simulink model "MdXX_Rsp"  (R2018b)
settings: Solver=FixedStepDiscrete  StartTime=0.0  StopTime=10.0  FixedStep=0.01  RelTol=1e-3
settings Model: Creator=sn2xws  LastModifiedBy=sn2xws
settings DataIOCC: SaveFormat=StructureWithTime
settings OptimizationCC: DefaultParameterBehavior=Inlined  EnhancedBackFolding=on  PassReuseOutputArgsAs=Individual arguments  ZeroExternalMemoryAtStartup=off  ZeroInternalMemoryAtStartup=off  OptimizeBlockOrder=speed  DifferentSizesBufferReuse=on  OptimizationCustomize=off
settings DebuggingCC: ParameterTunabilityLossMsg=error
settings ModelReferenceCC: ModelReferenceNumInstancesAllowed=Single
settings SFSimCC: MATLABDynamicMemAlloc=off
settings RTWCC: SystemTargetFile=autosar.tlc  GenCodeOnly=on  TemplateMakefile=ert_default_tmf  Description=AUTOSAR  GenerateReport=on  IncludeHyperlinkInReport=on  LaunchReport=on  GenerateTraceInfo=on  GenerateTraceReport=on  GenerateTraceReportSl=on  GenerateTraceReportSf=on  GenerateTraceReportEml=on
settings CodeAppCC: ForceParamTrailComments=on  IgnoreCustomStorageClasses=off  OperatorAnnotations=on  SimulinkDataObjDesc=on  SFDataObjDesc=on  InsertBlockDesc=on
settings STFCustomTargetCC: TargetLangStandard=C99 (ISO)  MultiwordLength=256  ParMdlRefBuildCompliant=on  CompOptLevelCompliant=on  IncludeMdlTerminateFcn=off  CombineOutputUpdateFcns=on  SuppressErrorStatus=on  ERTCustomFileBanners=on  SupportNonFinite=off  SupportComplex=off  SupportContinuousTime=off  SupportNonInlinedSFcns=off  RemoveResetFunc=on  MATLABClassNameForMDSCustomization=Simulink.SoftwareTarget.ERTCustomization  AutosarCompliant=on  UseToolchainInfoCompliant=on  LookupTableObjectStructAxisOrder=2,1,3,4,...  LUTObjectStructOrderEvenSpacing=Size,Table,Breakpoints  SystemTargetFile=autosar.tlc
settings ERTTargetCC: TargetLangStandard=C99 (ISO)  ConcurrentExecutionCompliant=off  IncludeMdlTerminateFcn=off  SuppressErrorStatus=on  SupportNonFinite=off  SupportComplex=off  ModelStepFunctionPrototypeControlCompliant=off  CPPClassGenCompliant=off  AutosarCompliant=on  LookupTableObjectStructAxisOrder=2,1,3,4,...  LUTObjectStructOrderEvenSpacing=Size,Table,Breakpoints  InlinedParameterPlacement=NonHierarchical  ERTCustomFileTemplate=example_file_process.tlc

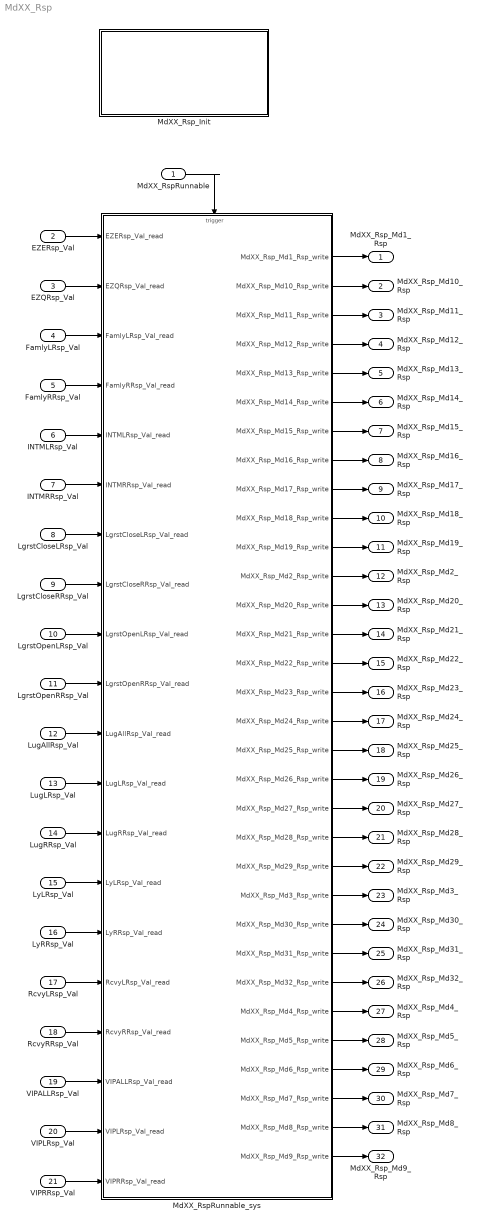
== system MdXX_Rsp ==
  MdXX_RspRunnable : Inport  SampleTime=0.01  OutputFunctionCall=on
  EZERsp_Val : Inport  Port=2  OutDataTypeStr=Enum: MdRspLocal1  PortDimensions=1
  EZQRsp_Val : Inport  Port=3  OutDataTypeStr=Enum: MdRspLocal1  PortDimensions=1
  FamlyLRsp_Val : Inport  Port=4  OutDataTypeStr=Enum: MdRspLocal1  PortDimensions=1
  FamlyRRsp_Val : Inport  Port=5  OutDataTypeStr=Enum: MdRspLocal1  PortDimensions=1
  INTMLRsp_Val : Inport  Port=6  OutDataTypeStr=Enum: MdRspLocal1  PortDimensions=1
  INTMRRsp_Val : Inport  Port=7  OutDataTypeStr=Enum: MdRspLocal1  PortDimensions=1
  LgrstCloseLRsp_Val : Inport  Port=8  OutDataTypeStr=Enum: MdRspLocal1  PortDimensions=1
  LgrstCloseRRsp_Val : Inport  Port=9  OutDataTypeStr=Enum: MdRspLocal1  PortDimensions=1
  LgrstOpenLRsp_Val : Inport  Port=10  OutDataTypeStr=Enum: MdRspLocal1  PortDimensions=1
  LgrstOpenRRsp_Val : Inport  Port=11  OutDataTypeStr=Enum: MdRspLocal1  PortDimensions=1
  LugAllRsp_Val : Inport  Port=12  OutDataTypeStr=Enum: MdRspLocal1  PortDimensions=1
  LugLRsp_Val : Inport  Port=13  OutDataTypeStr=Enum: MdRspLocal1  PortDimensions=1
  LugRRsp_Val : Inport  Port=14  OutDataTypeStr=Enum: MdRspLocal1  PortDimensions=1
  LyLRsp_Val : Inport  Port=15  OutDataTypeStr=Enum: MdRspLocal1  PortDimensions=1
  LyRRsp_Val : Inport  Port=16  OutDataTypeStr=Enum: MdRspLocal1  PortDimensions=1
  RcvyLRsp_Val : Inport  Port=17  OutDataTypeStr=Enum: MdRspLocal1  PortDimensions=1
  RcvyRRsp_Val : Inport  Port=18  OutDataTypeStr=Enum: MdRspLocal1  PortDimensions=1
  VIPALLRsp_Val : Inport  Port=19  OutDataTypeStr=Enum: MdRspLocal1  PortDimensions=1
  VIPLRsp_Val : Inport  Port=20  OutDataTypeStr=Enum: MdRspLocal1  PortDimensions=1
  VIPRRsp_Val : Inport  Port=21  OutDataTypeStr=Enum: MdRspLocal1  PortDimensions=1
  MdXX_RspRunnable_sys : Subsystem
  MdXX_Rsp_Init : Subsystem
  MdXX_Rsp_Md1_Rsp : Outport  OutDataTypeStr=Enum: MdRspLocal1  PortDimensions=1
  MdXX_Rsp_Md10_Rsp : Outport  Port=2  OutDataTypeStr=Enum: MdRspLocal1  PortDimensions=1
  MdXX_Rsp_Md11_Rsp : Outport  Port=3  OutDataTypeStr=Enum: MdRspLocal1  PortDimensions=1
  MdXX_Rsp_Md12_Rsp : Outport  Port=4  OutDataTypeStr=Enum: MdRspLocal1  PortDimensions=1
  MdXX_Rsp_Md13_Rsp : Outport  Port=5  OutDataTypeStr=Enum: MdRspLocal1  PortDimensions=1
  MdXX_Rsp_Md14_Rsp : Outport  Port=6  OutDataTypeStr=Enum: MdRspLocal1  PortDimensions=1
  MdXX_Rsp_Md15_Rsp : Outport  Port=7  OutDataTypeStr=Enum: MdRspLocal1  PortDimensions=1
  MdXX_Rsp_Md16_Rsp : Outport  Port=8  OutDataTypeStr=Enum: MdRspLocal1  PortDimensions=1
  MdXX_Rsp_Md17_Rsp : Outport  Port=9  OutDataTypeStr=Enum: MdRspLocal1  PortDimensions=1
  MdXX_Rsp_Md18_Rsp : Outport  Port=10  OutDataTypeStr=Enum: MdRspLocal1  PortDimensions=1
  MdXX_Rsp_Md19_Rsp : Outport  Port=11  OutDataTypeStr=Enum: MdRspLocal1  PortDimensions=1
  MdXX_Rsp_Md2_Rsp : Outport  Port=12  OutDataTypeStr=Enum: MdRspLocal1  PortDimensions=1
  MdXX_Rsp_Md20_Rsp : Outport  Port=13  OutDataTypeStr=Enum: MdRspLocal1  PortDimensions=1
  MdXX_Rsp_Md21_Rsp : Outport  Port=14  OutDataTypeStr=Enum: MdRspLocal1  PortDimensions=1
  MdXX_Rsp_Md22_Rsp : Outport  Port=15  OutDataTypeStr=Enum: MdRspLocal1  PortDimensions=1
  MdXX_Rsp_Md23_Rsp : Outport  Port=16  OutDataTypeStr=Enum: MdRspLocal1  PortDimensions=1
  MdXX_Rsp_Md24_Rsp : Outport  Port=17  OutDataTypeStr=Enum: MdRspLocal1  PortDimensions=1
  MdXX_Rsp_Md25_Rsp : Outport  Port=18  OutDataTypeStr=Enum: MdRspLocal1  PortDimensions=1
  MdXX_Rsp_Md26_Rsp : Outport  Port=19  OutDataTypeStr=Enum: MdRspLocal1  PortDimensions=1
  MdXX_Rsp_Md27_Rsp : Outport  Port=20  OutDataTypeStr=Enum: MdRspLocal1  PortDimensions=1
  MdXX_Rsp_Md28_Rsp : Outport  Port=21  OutDataTypeStr=Enum: MdRspLocal1  PortDimensions=1
  MdXX_Rsp_Md29_Rsp : Outport  Port=22  OutDataTypeStr=Enum: MdRspLocal1  PortDimensions=1
  MdXX_Rsp_Md3_Rsp : Outport  Port=23  OutDataTypeStr=Enum: MdRspLocal1  PortDimensions=1
  MdXX_Rsp_Md30_Rsp : Outport  Port=24  OutDataTypeStr=Enum: MdRspLocal1  PortDimensions=1
  MdXX_Rsp_Md31_Rsp : Outport  Port=25  OutDataTypeStr=Enum: MdRspLocal1  PortDimensions=1
  MdXX_Rsp_Md32_Rsp : Outport  Port=26  OutDataTypeStr=Enum: MdRspLocal1  PortDimensions=1
  MdXX_Rsp_Md4_Rsp : Outport  Port=27  OutDataTypeStr=Enum: MdRspLocal1  PortDimensions=1
  MdXX_Rsp_Md5_Rsp : Outport  Port=28  OutDataTypeStr=Enum: MdRspLocal1  PortDimensions=1
  MdXX_Rsp_Md6_Rsp : Outport  Port=29  OutDataTypeStr=Enum: MdRspLocal1  PortDimensions=1
  MdXX_Rsp_Md7_Rsp : Outport  Port=30  OutDataTypeStr=Enum: MdRspLocal1  PortDimensions=1
  MdXX_Rsp_Md8_Rsp : Outport  Port=31  OutDataTypeStr=Enum: MdRspLocal1  PortDimensions=1
  MdXX_Rsp_Md9_Rsp : Outport  Port=32  OutDataTypeStr=Enum: MdRspLocal1  PortDimensions=1
  wires:
  EZERsp_Val/1 -> MdXX_RspRunnable_sys/1(EZERsp_Val_read)
  EZQRsp_Val/1 -> MdXX_RspRunnable_sys/2(EZQRsp_Val_read)
  FamlyLRsp_Val/1 -> MdXX_RspRunnable_sys/3(FamlyLRsp_Val_read)
  FamlyRRsp_Val/1 -> MdXX_RspRunnable_sys/4(FamlyRRsp_Val_read)
  INTMLRsp_Val/1 -> MdXX_RspRunnable_sys/5(INTMLRsp_Val_read)
  INTMRRsp_Val/1 -> MdXX_RspRunnable_sys/6(INTMRRsp_Val_read)
  LgrstCloseLRsp_Val/1 -> MdXX_RspRunnable_sys/7(LgrstCloseLRsp_Val_read)
  LgrstCloseRRsp_Val/1 -> MdXX_RspRunnable_sys/8(LgrstCloseRRsp_Val_read)
  LgrstOpenLRsp_Val/1 -> MdXX_RspRunnable_sys/9(LgrstOpenLRsp_Val_read)
  LgrstOpenRRsp_Val/1 -> MdXX_RspRunnable_sys/10(LgrstOpenRRsp_Val_read)
  LugAllRsp_Val/1 -> MdXX_RspRunnable_sys/11(LugAllRsp_Val_read)
  LugLRsp_Val/1 -> MdXX_RspRunnable_sys/12(LugLRsp_Val_read)
  LugRRsp_Val/1 -> MdXX_RspRunnable_sys/13(LugRRsp_Val_read)
  LyLRsp_Val/1 -> MdXX_RspRunnable_sys/14(LyLRsp_Val_read)
  LyRRsp_Val/1 -> MdXX_RspRunnable_sys/15(LyRRsp_Val_read)
  RcvyLRsp_Val/1 -> MdXX_RspRunnable_sys/16(RcvyLRsp_Val_read)
  RcvyRRsp_Val/1 -> MdXX_RspRunnable_sys/17(RcvyRRsp_Val_read)
  VIPALLRsp_Val/1 -> MdXX_RspRunnable_sys/18(VIPALLRsp_Val_read)
  VIPLRsp_Val/1 -> MdXX_RspRunnable_sys/19(VIPLRsp_Val_read)
  VIPRRsp_Val/1 -> MdXX_RspRunnable_sys/20(VIPRRsp_Val_read)
  MdXX_RspRunnable_sys/1(MdXX_Rsp_Md1_Rsp_write) -> MdXX_Rsp_Md1_Rsp/1
  MdXX_RspRunnable_sys/2(MdXX_Rsp_Md10_Rsp_write) -> MdXX_Rsp_Md10_Rsp/1
  MdXX_RspRunnable_sys/3(MdXX_Rsp_Md11_Rsp_write) -> MdXX_Rsp_Md11_Rsp/1
  MdXX_RspRunnable_sys/4(MdXX_Rsp_Md12_Rsp_write) -> MdXX_Rsp_Md12_Rsp/1
  MdXX_RspRunnable_sys/5(MdXX_Rsp_Md13_Rsp_write) -> MdXX_Rsp_Md13_Rsp/1
  MdXX_RspRunnable_sys/6(MdXX_Rsp_Md14_Rsp_write) -> MdXX_Rsp_Md14_Rsp/1
  MdXX_RspRunnable_sys/7(MdXX_Rsp_Md15_Rsp_write) -> MdXX_Rsp_Md15_Rsp/1
  MdXX_RspRunnable_sys/8(MdXX_Rsp_Md16_Rsp_write) -> MdXX_Rsp_Md16_Rsp/1
  MdXX_RspRunnable_sys/9(MdXX_Rsp_Md17_Rsp_write) -> MdXX_Rsp_Md17_Rsp/1
  MdXX_RspRunnable_sys/10(MdXX_Rsp_Md18_Rsp_write) -> MdXX_Rsp_Md18_Rsp/1
  MdXX_RspRunnable_sys/11(MdXX_Rsp_Md19_Rsp_write) -> MdXX_Rsp_Md19_Rsp/1
  MdXX_RspRunnable_sys/12(MdXX_Rsp_Md2_Rsp_write) -> MdXX_Rsp_Md2_Rsp/1
  MdXX_RspRunnable_sys/13(MdXX_Rsp_Md20_Rsp_write) -> MdXX_Rsp_Md20_Rsp/1
  MdXX_RspRunnable_sys/14(MdXX_Rsp_Md21_Rsp_write) -> MdXX_Rsp_Md21_Rsp/1
  MdXX_RspRunnable_sys/15(MdXX_Rsp_Md22_Rsp_write) -> MdXX_Rsp_Md22_Rsp/1
  MdXX_RspRunnable_sys/16(MdXX_Rsp_Md23_Rsp_write) -> MdXX_Rsp_Md23_Rsp/1
  MdXX_RspRunnable_sys/17(MdXX_Rsp_Md24_Rsp_write) -> MdXX_Rsp_Md24_Rsp/1
  MdXX_RspRunnable_sys/18(MdXX_Rsp_Md25_Rsp_write) -> MdXX_Rsp_Md25_Rsp/1
  MdXX_RspRunnable_sys/19(MdXX_Rsp_Md26_Rsp_write) -> MdXX_Rsp_Md26_Rsp/1
  MdXX_RspRunnable_sys/20(MdXX_Rsp_Md27_Rsp_write) -> MdXX_Rsp_Md27_Rsp/1
  MdXX_RspRunnable_sys/21(MdXX_Rsp_Md28_Rsp_write) -> MdXX_Rsp_Md28_Rsp/1
  MdXX_RspRunnable_sys/22(MdXX_Rsp_Md29_Rsp_write) -> MdXX_Rsp_Md29_Rsp/1
  MdXX_RspRunnable_sys/23(MdXX_Rsp_Md3_Rsp_write) -> MdXX_Rsp_Md3_Rsp/1
  MdXX_RspRunnable_sys/24(MdXX_Rsp_Md30_Rsp_write) -> MdXX_Rsp_Md30_Rsp/1
  MdXX_RspRunnable_sys/25(MdXX_Rsp_Md31_Rsp_write) -> MdXX_Rsp_Md31_Rsp/1
  MdXX_RspRunnable_sys/26(MdXX_Rsp_Md32_Rsp_write) -> MdXX_Rsp_Md32_Rsp/1
  MdXX_RspRunnable_sys/27(MdXX_Rsp_Md4_Rsp_write) -> MdXX_Rsp_Md4_Rsp/1
  MdXX_RspRunnable_sys/28(MdXX_Rsp_Md5_Rsp_write) -> MdXX_Rsp_Md5_Rsp/1
  MdXX_RspRunnable_sys/29(MdXX_Rsp_Md6_Rsp_write) -> MdXX_Rsp_Md6_Rsp/1
  MdXX_RspRunnable_sys/30(MdXX_Rsp_Md7_Rsp_write) -> MdXX_Rsp_Md7_Rsp/1
  MdXX_RspRunnable_sys/31(MdXX_Rsp_Md8_Rsp_write) -> MdXX_Rsp_Md8_Rsp/1
  MdXX_RspRunnable_sys/32(MdXX_Rsp_Md9_Rsp_write) -> MdXX_Rsp_Md9_Rsp/1
  MdXX_RspRunnable/1 -> MdXX_RspRunnable_sys/Trigger

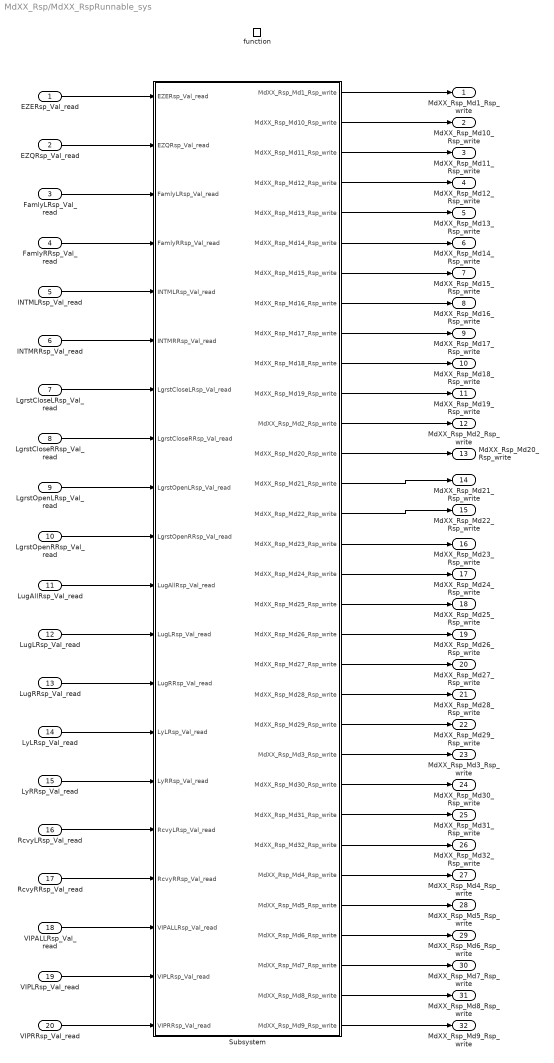
== system MdXX_Rsp/MdXX_RspRunnable_sys ==
  EZERsp_Val_read : Inport
  EZQRsp_Val_read : Inport  Port=2
  FamlyLRsp_Val_read : Inport  Port=3
  FamlyRRsp_Val_read : Inport  Port=4
  INTMLRsp_Val_read : Inport  Port=5
  INTMRRsp_Val_read : Inport  Port=6
  LgrstCloseLRsp_Val_read : Inport  Port=7
  LgrstCloseRRsp_Val_read : Inport  Port=8
  LgrstOpenLRsp_Val_read : Inport  Port=9
  LgrstOpenRRsp_Val_read : Inport  Port=10
  LugAllRsp_Val_read : Inport  Port=11
  LugLRsp_Val_read : Inport  Port=12
  LugRRsp_Val_read : Inport  Port=13
  LyLRsp_Val_read : Inport  Port=14
  LyRRsp_Val_read : Inport  Port=15
  RcvyLRsp_Val_read : Inport  Port=16
  RcvyRRsp_Val_read : Inport  Port=17
  VIPALLRsp_Val_read : Inport  Port=18
  VIPLRsp_Val_read : Inport  Port=19
  VIPRRsp_Val_read : Inport  Port=20
  function : TriggerPort  TriggerType=function-call  VariantControl=(inherit)  SampleTimeType=periodic  SampleTime=-1
  Subsystem : Subsystem
  MdXX_Rsp_Md1_Rsp_write : Outport
      settings: EnsureOutportIsVirtual=on
  MdXX_Rsp_Md10_Rsp_write : Outport  Port=2
      settings: EnsureOutportIsVirtual=on
  MdXX_Rsp_Md11_Rsp_write : Outport  Port=3
      settings: EnsureOutportIsVirtual=on
  MdXX_Rsp_Md12_Rsp_write : Outport  Port=4
      settings: EnsureOutportIsVirtual=on
  MdXX_Rsp_Md13_Rsp_write : Outport  Port=5
      settings: EnsureOutportIsVirtual=on
  MdXX_Rsp_Md14_Rsp_write : Outport  Port=6
      settings: EnsureOutportIsVirtual=on
  MdXX_Rsp_Md15_Rsp_write : Outport  Port=7
      settings: EnsureOutportIsVirtual=on
  MdXX_Rsp_Md16_Rsp_write : Outport  Port=8
      settings: EnsureOutportIsVirtual=on
  MdXX_Rsp_Md17_Rsp_write : Outport  Port=9
      settings: EnsureOutportIsVirtual=on
  MdXX_Rsp_Md18_Rsp_write : Outport  Port=10
      settings: EnsureOutportIsVirtual=on
  MdXX_Rsp_Md19_Rsp_write : Outport  Port=11
      settings: EnsureOutportIsVirtual=on
  MdXX_Rsp_Md2_Rsp_write : Outport  Port=12
      settings: EnsureOutportIsVirtual=on
  MdXX_Rsp_Md20_Rsp_write : Outport  Port=13
      settings: EnsureOutportIsVirtual=on
  MdXX_Rsp_Md21_Rsp_write : Outport  Port=14
      settings: EnsureOutportIsVirtual=on
  MdXX_Rsp_Md22_Rsp_write : Outport  Port=15
      settings: EnsureOutportIsVirtual=on
  MdXX_Rsp_Md23_Rsp_write : Outport  Port=16
      settings: EnsureOutportIsVirtual=on
  MdXX_Rsp_Md24_Rsp_write : Outport  Port=17
      settings: EnsureOutportIsVirtual=on
  MdXX_Rsp_Md25_Rsp_write : Outport  Port=18
      settings: EnsureOutportIsVirtual=on
  MdXX_Rsp_Md26_Rsp_write : Outport  Port=19
      settings: EnsureOutportIsVirtual=on
  MdXX_Rsp_Md27_Rsp_write : Outport  Port=20
      settings: EnsureOutportIsVirtual=on
  MdXX_Rsp_Md28_Rsp_write : Outport  Port=21
      settings: EnsureOutportIsVirtual=on
  MdXX_Rsp_Md29_Rsp_write : Outport  Port=22
      settings: EnsureOutportIsVirtual=on
  MdXX_Rsp_Md3_Rsp_write : Outport  Port=23
      settings: EnsureOutportIsVirtual=on
  MdXX_Rsp_Md30_Rsp_write : Outport  Port=24
      settings: EnsureOutportIsVirtual=on
  MdXX_Rsp_Md31_Rsp_write : Outport  Port=25
      settings: EnsureOutportIsVirtual=on
  MdXX_Rsp_Md32_Rsp_write : Outport  Port=26
      settings: EnsureOutportIsVirtual=on
  MdXX_Rsp_Md4_Rsp_write : Outport  Port=27
      settings: EnsureOutportIsVirtual=on
  MdXX_Rsp_Md5_Rsp_write : Outport  Port=28
      settings: EnsureOutportIsVirtual=on
  MdXX_Rsp_Md6_Rsp_write : Outport  Port=29
      settings: EnsureOutportIsVirtual=on
  MdXX_Rsp_Md7_Rsp_write : Outport  Port=30
      settings: EnsureOutportIsVirtual=on
  MdXX_Rsp_Md8_Rsp_write : Outport  Port=31
      settings: EnsureOutportIsVirtual=on
  MdXX_Rsp_Md9_Rsp_write : Outport  Port=32
      settings: EnsureOutportIsVirtual=on
  wires:
  EZERsp_Val_read/1 -> Subsystem/1(EZERsp_Val_read)
  EZQRsp_Val_read/1 -> Subsystem/2(EZQRsp_Val_read)
  FamlyLRsp_Val_read/1 -> Subsystem/3(FamlyLRsp_Val_read)
  FamlyRRsp_Val_read/1 -> Subsystem/4(FamlyRRsp_Val_read)
  INTMLRsp_Val_read/1 -> Subsystem/5(INTMLRsp_Val_read)
  INTMRRsp_Val_read/1 -> Subsystem/6(INTMRRsp_Val_read)
  LgrstCloseLRsp_Val_read/1 -> Subsystem/7(LgrstCloseLRsp_Val_read)
  LgrstCloseRRsp_Val_read/1 -> Subsystem/8(LgrstCloseRRsp_Val_read)
  LgrstOpenLRsp_Val_read/1 -> Subsystem/9(LgrstOpenLRsp_Val_read)
  LgrstOpenRRsp_Val_read/1 -> Subsystem/10(LgrstOpenRRsp_Val_read)
  LugAllRsp_Val_read/1 -> Subsystem/11(LugAllRsp_Val_read)
  LugLRsp_Val_read/1 -> Subsystem/12(LugLRsp_Val_read)
  LugRRsp_Val_read/1 -> Subsystem/13(LugRRsp_Val_read)
  LyLRsp_Val_read/1 -> Subsystem/14(LyLRsp_Val_read)
  LyRRsp_Val_read/1 -> Subsystem/15(LyRRsp_Val_read)
  RcvyLRsp_Val_read/1 -> Subsystem/16(RcvyLRsp_Val_read)
  RcvyRRsp_Val_read/1 -> Subsystem/17(RcvyRRsp_Val_read)
  VIPALLRsp_Val_read/1 -> Subsystem/18(VIPALLRsp_Val_read)
  VIPLRsp_Val_read/1 -> Subsystem/19(VIPLRsp_Val_read)
  VIPRRsp_Val_read/1 -> Subsystem/20(VIPRRsp_Val_read)
  Subsystem/1(MdXX_Rsp_Md1_Rsp_write) -> MdXX_Rsp_Md1_Rsp_write/1
  Subsystem/2(MdXX_Rsp_Md10_Rsp_write) -> MdXX_Rsp_Md10_Rsp_write/1
  Subsystem/3(MdXX_Rsp_Md11_Rsp_write) -> MdXX_Rsp_Md11_Rsp_write/1
  Subsystem/4(MdXX_Rsp_Md12_Rsp_write) -> MdXX_Rsp_Md12_Rsp_write/1
  Subsystem/5(MdXX_Rsp_Md13_Rsp_write) -> MdXX_Rsp_Md13_Rsp_write/1
  Subsystem/6(MdXX_Rsp_Md14_Rsp_write) -> MdXX_Rsp_Md14_Rsp_write/1
  Subsystem/7(MdXX_Rsp_Md15_Rsp_write) -> MdXX_Rsp_Md15_Rsp_write/1
  Subsystem/8(MdXX_Rsp_Md16_Rsp_write) -> MdXX_Rsp_Md16_Rsp_write/1
  Subsystem/9(MdXX_Rsp_Md17_Rsp_write) -> MdXX_Rsp_Md17_Rsp_write/1
  Subsystem/10(MdXX_Rsp_Md18_Rsp_write) -> MdXX_Rsp_Md18_Rsp_write/1
  Subsystem/11(MdXX_Rsp_Md19_Rsp_write) -> MdXX_Rsp_Md19_Rsp_write/1
  Subsystem/12(MdXX_Rsp_Md2_Rsp_write) -> MdXX_Rsp_Md2_Rsp_write/1
  Subsystem/13(MdXX_Rsp_Md20_Rsp_write) -> MdXX_Rsp_Md20_Rsp_write/1
  Subsystem/14(MdXX_Rsp_Md21_Rsp_write) -> MdXX_Rsp_Md21_Rsp_write/1
  Subsystem/15(MdXX_Rsp_Md22_Rsp_write) -> MdXX_Rsp_Md22_Rsp_write/1
  Subsystem/16(MdXX_Rsp_Md23_Rsp_write) -> MdXX_Rsp_Md23_Rsp_write/1
  Subsystem/17(MdXX_Rsp_Md24_Rsp_write) -> MdXX_Rsp_Md24_Rsp_write/1
  Subsystem/18(MdXX_Rsp_Md25_Rsp_write) -> MdXX_Rsp_Md25_Rsp_write/1
  Subsystem/19(MdXX_Rsp_Md26_Rsp_write) -> MdXX_Rsp_Md26_Rsp_write/1
  Subsystem/20(MdXX_Rsp_Md27_Rsp_write) -> MdXX_Rsp_Md27_Rsp_write/1
  Subsystem/21(MdXX_Rsp_Md28_Rsp_write) -> MdXX_Rsp_Md28_Rsp_write/1
  Subsystem/22(MdXX_Rsp_Md29_Rsp_write) -> MdXX_Rsp_Md29_Rsp_write/1
  Subsystem/23(MdXX_Rsp_Md3_Rsp_write) -> MdXX_Rsp_Md3_Rsp_write/1
  Subsystem/24(MdXX_Rsp_Md30_Rsp_write) -> MdXX_Rsp_Md30_Rsp_write/1
  Subsystem/25(MdXX_Rsp_Md31_Rsp_write) -> MdXX_Rsp_Md31_Rsp_write/1
  Subsystem/26(MdXX_Rsp_Md32_Rsp_write) -> MdXX_Rsp_Md32_Rsp_write/1
  Subsystem/27(MdXX_Rsp_Md4_Rsp_write) -> MdXX_Rsp_Md4_Rsp_write/1
  Subsystem/28(MdXX_Rsp_Md5_Rsp_write) -> MdXX_Rsp_Md5_Rsp_write/1
  Subsystem/29(MdXX_Rsp_Md6_Rsp_write) -> MdXX_Rsp_Md6_Rsp_write/1
  Subsystem/30(MdXX_Rsp_Md7_Rsp_write) -> MdXX_Rsp_Md7_Rsp_write/1
  Subsystem/31(MdXX_Rsp_Md8_Rsp_write) -> MdXX_Rsp_Md8_Rsp_write/1
  Subsystem/32(MdXX_Rsp_Md9_Rsp_write) -> MdXX_Rsp_Md9_Rsp_write/1

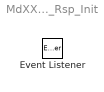
== system MdXX_Rsp/MdXX_Rsp_Init ==
  Event Listener : EventListener  EventName=reset

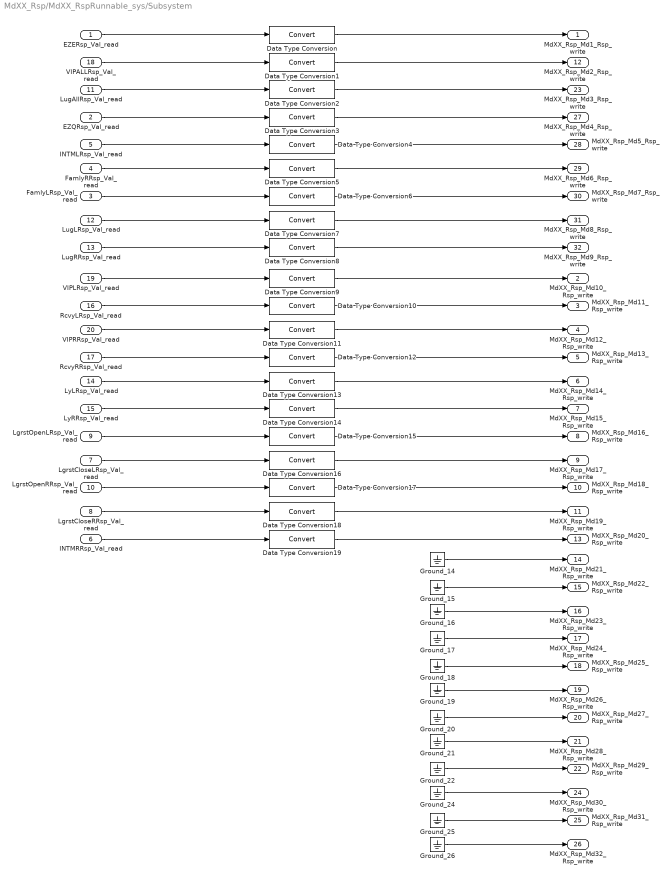
== system MdXX_Rsp/MdXX_RspRunnable_sys/Subsystem ==
  EZERsp_Val_read : Inport
  EZQRsp_Val_read : Inport  Port=2
  FamlyLRsp_Val_read : Inport  Port=3
  FamlyRRsp_Val_read : Inport  Port=4
  INTMLRsp_Val_read : Inport  Port=5
  INTMRRsp_Val_read : Inport  Port=6
  LgrstCloseLRsp_Val_read : Inport  Port=7
  LgrstCloseRRsp_Val_read : Inport  Port=8
  LgrstOpenLRsp_Val_read : Inport  Port=9
  LgrstOpenRRsp_Val_read : Inport  Port=10
  LugAllRsp_Val_read : Inport  Port=11
  LugLRsp_Val_read : Inport  Port=12
  LugRRsp_Val_read : Inport  Port=13
  LyLRsp_Val_read : Inport  Port=14
  LyRRsp_Val_read : Inport  Port=15
  RcvyLRsp_Val_read : Inport  Port=16
  RcvyRRsp_Val_read : Inport  Port=17
  VIPALLRsp_Val_read : Inport  Port=18
  VIPLRsp_Val_read : Inport  Port=19
  VIPRRsp_Val_read : Inport  Port=20
  Data Type Conversion{,1..19} (20 alike) : DataTypeConversion
  Ground_{14..22,24..26} (12 alike) : Ground
  MdXX_Rsp_Md1_Rsp_write : Outport
      settings: EnsureOutportIsVirtual=on
  MdXX_Rsp_Md10_Rsp_write : Outport  Port=2
      settings: EnsureOutportIsVirtual=on
  MdXX_Rsp_Md11_Rsp_write : Outport  Port=3
      settings: EnsureOutportIsVirtual=on
  MdXX_Rsp_Md12_Rsp_write : Outport  Port=4
      settings: EnsureOutportIsVirtual=on
  MdXX_Rsp_Md13_Rsp_write : Outport  Port=5
      settings: EnsureOutportIsVirtual=on
  MdXX_Rsp_Md14_Rsp_write : Outport  Port=6
      settings: EnsureOutportIsVirtual=on
  MdXX_Rsp_Md15_Rsp_write : Outport  Port=7
      settings: EnsureOutportIsVirtual=on
  MdXX_Rsp_Md16_Rsp_write : Outport  Port=8
      settings: EnsureOutportIsVirtual=on
  MdXX_Rsp_Md17_Rsp_write : Outport  Port=9
      settings: EnsureOutportIsVirtual=on
  MdXX_Rsp_Md18_Rsp_write : Outport  Port=10
      settings: EnsureOutportIsVirtual=on
  MdXX_Rsp_Md19_Rsp_write : Outport  Port=11
      settings: EnsureOutportIsVirtual=on
  MdXX_Rsp_Md2_Rsp_write : Outport  Port=12
      settings: EnsureOutportIsVirtual=on
  MdXX_Rsp_Md20_Rsp_write : Outport  Port=13
      settings: EnsureOutportIsVirtual=on
  MdXX_Rsp_Md21_Rsp_write : Outport  Port=14
      settings: EnsureOutportIsVirtual=on
  MdXX_Rsp_Md22_Rsp_write : Outport  Port=15
      settings: EnsureOutportIsVirtual=on
  MdXX_Rsp_Md23_Rsp_write : Outport  Port=16
      settings: EnsureOutportIsVirtual=on
  MdXX_Rsp_Md24_Rsp_write : Outport  Port=17
      settings: EnsureOutportIsVirtual=on
  MdXX_Rsp_Md25_Rsp_write : Outport  Port=18
      settings: EnsureOutportIsVirtual=on
  MdXX_Rsp_Md26_Rsp_write : Outport  Port=19
      settings: EnsureOutportIsVirtual=on
  MdXX_Rsp_Md27_Rsp_write : Outport  Port=20
      settings: EnsureOutportIsVirtual=on
  MdXX_Rsp_Md28_Rsp_write : Outport  Port=21
      settings: EnsureOutportIsVirtual=on
  MdXX_Rsp_Md29_Rsp_write : Outport  Port=22
      settings: EnsureOutportIsVirtual=on
  MdXX_Rsp_Md3_Rsp_write : Outport  Port=23
      settings: EnsureOutportIsVirtual=on
  MdXX_Rsp_Md30_Rsp_write : Outport  Port=24
      settings: EnsureOutportIsVirtual=on
  MdXX_Rsp_Md31_Rsp_write : Outport  Port=25
      settings: EnsureOutportIsVirtual=on
  MdXX_Rsp_Md32_Rsp_write : Outport  Port=26
      settings: EnsureOutportIsVirtual=on
  MdXX_Rsp_Md4_Rsp_write : Outport  Port=27
      settings: EnsureOutportIsVirtual=on
  MdXX_Rsp_Md5_Rsp_write : Outport  Port=28
      settings: EnsureOutportIsVirtual=on
  MdXX_Rsp_Md6_Rsp_write : Outport  Port=29
      settings: EnsureOutportIsVirtual=on
  MdXX_Rsp_Md7_Rsp_write : Outport  Port=30
      settings: EnsureOutportIsVirtual=on
  MdXX_Rsp_Md8_Rsp_write : Outport  Port=31
      settings: EnsureOutportIsVirtual=on
  MdXX_Rsp_Md9_Rsp_write : Outport  Port=32
      settings: EnsureOutportIsVirtual=on
  wires:
  Ground_16/1 -> MdXX_Rsp_Md23_Rsp_write/1
  Ground_22/1 -> MdXX_Rsp_Md29_Rsp_write/1
  Ground_26/1 -> MdXX_Rsp_Md32_Rsp_write/1
  Ground_15/1 -> MdXX_Rsp_Md22_Rsp_write/1
  VIPALLRsp_Val_read/1 -> Data Type Conversion1/1
  Ground_21/1 -> MdXX_Rsp_Md28_Rsp_write/1
  Ground_17/1 -> MdXX_Rsp_Md24_Rsp_write/1
  EZERsp_Val_read/1 -> Data Type Conversion/1
  Ground_14/1 -> MdXX_Rsp_Md21_Rsp_write/1
  Ground_18/1 -> MdXX_Rsp_Md25_Rsp_write/1
  Ground_25/1 -> MdXX_Rsp_Md31_Rsp_write/1
  Ground_24/1 -> MdXX_Rsp_Md30_Rsp_write/1
  Ground_20/1 -> MdXX_Rsp_Md27_Rsp_write/1
  Ground_19/1 -> MdXX_Rsp_Md26_Rsp_write/1
  LugAllRsp_Val_read/1 -> Data Type Conversion2/1
  INTMLRsp_Val_read/1 -> Data Type Conversion4/1
  FamlyRRsp_Val_read/1 -> Data Type Conversion5/1
  FamlyLRsp_Val_read/1 -> Data Type Conversion6/1
  LugRRsp_Val_read/1 -> Data Type Conversion8/1
  LugLRsp_Val_read/1 -> Data Type Conversion7/1
  VIPLRsp_Val_read/1 -> Data Type Conversion9/1
  RcvyLRsp_Val_read/1 -> Data Type Conversion10/1
  VIPRRsp_Val_read/1 -> Data Type Conversion11/1
  RcvyRRsp_Val_read/1 -> Data Type Conversion12/1
  LyLRsp_Val_read/1 -> Data Type Conversion13/1
  LyRRsp_Val_read/1 -> Data Type Conversion14/1
  LgrstOpenLRsp_Val_read/1 -> Data Type Conversion15/1
  LgrstCloseLRsp_Val_read/1 -> Data Type Conversion16/1
  LgrstOpenRRsp_Val_read/1 -> Data Type Conversion17/1
  LgrstCloseRRsp_Val_read/1 -> Data Type Conversion18/1
  INTMRRsp_Val_read/1 -> Data Type Conversion19/1
  EZQRsp_Val_read/1 -> Data Type Conversion3/1
  Data Type Conversion/1 -> MdXX_Rsp_Md1_Rsp_write/1
  Data Type Conversion1/1 -> MdXX_Rsp_Md2_Rsp_write/1
  Data Type Conversion2/1 -> MdXX_Rsp_Md3_Rsp_write/1
  Data Type Conversion3/1 -> MdXX_Rsp_Md4_Rsp_write/1
  Data Type Conversion4/1 -> MdXX_Rsp_Md5_Rsp_write/1
  Data Type Conversion5/1 -> MdXX_Rsp_Md6_Rsp_write/1
  Data Type Conversion6/1 -> MdXX_Rsp_Md7_Rsp_write/1
  Data Type Conversion7/1 -> MdXX_Rsp_Md8_Rsp_write/1
  Data Type Conversion8/1 -> MdXX_Rsp_Md9_Rsp_write/1
  Data Type Conversion9/1 -> MdXX_Rsp_Md10_Rsp_write/1
  Data Type Conversion10/1 -> MdXX_Rsp_Md11_Rsp_write/1
  Data Type Conversion11/1 -> MdXX_Rsp_Md12_Rsp_write/1
  Data Type Conversion12/1 -> MdXX_Rsp_Md13_Rsp_write/1
  Data Type Conversion13/1 -> MdXX_Rsp_Md14_Rsp_write/1
  Data Type Conversion14/1 -> MdXX_Rsp_Md15_Rsp_write/1
  Data Type Conversion15/1 -> MdXX_Rsp_Md16_Rsp_write/1
  Data Type Conversion16/1 -> MdXX_Rsp_Md17_Rsp_write/1
  Data Type Conversion17/1 -> MdXX_Rsp_Md18_Rsp_write/1
  Data Type Conversion18/1 -> MdXX_Rsp_Md19_Rsp_write/1
  Data Type Conversion19/1 -> MdXX_Rsp_Md20_Rsp_write/1
